simulink model "HalfBridgeInverter"  (R2014a)
settings: Solver=ode45  StartTime=0.0  StopTime=0.1  RelTol=1e-3
libraries: powerlib x9
settings Model: Creator=ninad gaikawad  LastModifiedBy=ninad gaikawad

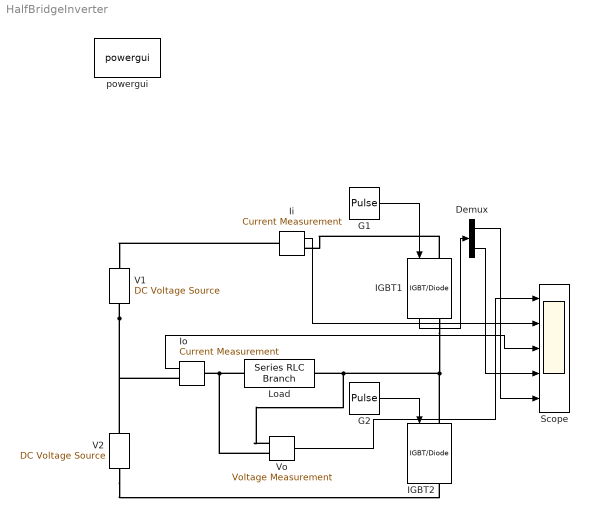
== system HalfBridgeInverter ==
  Demux : Demux  Outputs=2
  G1 : DiscretePulseGenerator  PulseType=Time based  Period=20*10^(-3)  PulseWidth=50
  G2 : DiscretePulseGenerator  PulseType=Time based  Period=20*10^(-3)  PulseWidth=50  PhaseDelay=0.01
  IGBT1 : powerlib/Power Electronics/IGBT//Diode  Ron=1e-3  Rs=1e5  Cs=inf  Measurements=on
  IGBT2 : powerlib/Power Electronics/IGBT//Diode  Ron=1e-3  Rs=1e5  Cs=inf  Measurements=on
  Ii : powerlib/Measurements/Current Measurement  PhasorSimulation=off  OutputType=Complex  PSBequivalent=0
  Io : powerlib/Measurements/Current Measurement  PhasorSimulation=off  OutputType=Complex  PSBequivalent=0
  Load : powerlib/Elements/Series RLC Branch  LConnTagsString=__new0  RConnTagsString=__new0  BranchType=R  Resistance=0.5  Inductance=0.01  SetiL0=off  InitialCurrent=0  Capacitance=1e-6  Setx0=off  InitialVoltage=0  Measurements=None
  Scope : Scope  NumInputPorts=5
      settings: TimeRange=5  YMin=-5~-5~-5~-5~-5  YMax=5~5~5~5~5
  V1 : powerlib/Electrical Sources/DC Voltage Source  Amplitude=125  Measurements=None
  V2 : powerlib/Electrical Sources/DC Voltage Source  Amplitude=125  Measurements=None
  Vo : powerlib/Measurements/Voltage Measurement  PhasorSimulation=off  OutputType=Complex  PSBequivalent=0
  powergui : powerlib/powergui  Priority=1  SimulationMode=Continuous  SolverType=Tustin  SampleTime=50e-6  frequency=60  SPID=off  DisableSnubberDevices=off  DisableRonSwitches=off  DisableVfSwitches=off  SwTol=0  Interpol=off  DisplayEquations=off  Ts=0  methode=off  frequencyindice=0  Pbase=100e6  ErrMax=1e-4  Iterations=50  UnitsV=kV  UnitsW=MW  FunctionMessages=off  echomessages=off  HookPort=off  EnableUseOfTLC=off  x0status=blocks  RestoreLinks=warning  ResistiveCurrentMeasurement=off  Frange=[0:2:500]  Ylog=off  Xlog=on  ShowGrid=off  save=off  variable=ZData  structure=0  ZoomFFT=off  StartTime=0.0  cycles=1  DisplayStyle=1  fundamental=60  FreqAxis=off  MaxFrequency=1000  frequencyindicesteady=1  RmsSteady=1  display=off
  wires:
  G2/1 -> IGBT2/1
  G1/1 -> IGBT1/1
  Vo/1 -> Scope/1
  Ii/1 -> Scope/2
  Io/1 -> Scope/3
  IGBT1/1 -> Demux/1
  Demux/1 -> Scope/5
  Demux/2 -> Scope/4
  connections:
  Ii/LConn1 -- V1/RConn1
  IGBT1/RConn1 -- IGBT2/LConn1 -- Vo/LConn1 -- Load/RConn1
  V1/LConn1 -- Io/RConn1 -- V2/RConn1
  V2/LConn1 -- IGBT2/RConn1
  IGBT1/LConn1 -- Ii/RConn1
  Load/LConn1 -- Vo/LConn2 -- Io/LConn1
